simulink model "Basic_DMT"  (R2014b)
settings: Solver=FixedStepDiscrete  SolverMode=SingleTasking  StartTime=0.0  StopTime=25e-6-14e-9*24  RelTol=1e-3
PreLoadFcn:
  | userName = getenv('UserName');
  | 
  | if strcmp(userName,'Tim')
  | cd C:\Users\Tim\Documents\GitHub\MA_1\Basic_DMT
  | else
  | cd C:\Users\Tim-UML\Documents\GitHub\MA_1\Basic_DMT
  | end
InitFcn:
  | userName = getenv('UserName');
  | 
  | if strcmp(userName,'Tim')
  | cd C:\Users\Tim\Documents\GitHub\MA_1\Basic_DMT
  | else
  | cd C:\Users\Tim-UML\Documents\GitHub\MA_1\Basic_DMT
  | end
values from neighbouring files (symbols this model uses):
  a0 = 0.21194908595403703    (= 0.211949085954)    [initScript.m]
  a1 = 0.576101828091926    (= 0.576101828092)    [initScript.m]
  a2 = a0    (= 0.211949085954)    [initScript.m]
  beta = 1    [initScript.m]
  bitPerSymb = 4    [initScript.m]
  chanDownFact = Tchan/SystemPeriod    [initScript.m]
  fftLen = 16    [initScript.m]
  fftLenActive = fftLenDMT    (= 32)    [initScript.m]
  fftLenDMT = 2*fftLen    (= 32)    [initScript.m]
  GI_Active = GI_LenDMT    (= 0)    [initScript.m]
  GI_Len = 0    [initScript.m]
  GI_LenDMT = 0    [initScript.m]
  M = log2(fftLen)    [initScript.m]
  sysgenSystemPeriod = 4e-9    (= 4e-09)    [initScript.m]
  SystemPeriod = 4e-9    (= 4e-09)    [initScript.m]
  upsampleFactor = 1    [initScript.m]
  usedSubCar = 14    [initScript.m]
undefined symbols (not defined in the file or in its folder): bitCount, get, modu_mode, Tb, Ts
libraries: xbsIndex_r4 x822, commdigbbndam3 x59, simulink x42, dspsigops x7, commrandsrc2 x6, dspbuff3 x4, dspxfrm3 x3, dspswit3 x2, commseqgen2 x1, dsparch4 x1, commutil2 x1, dspsnks4 x1
(part 8 of 10)

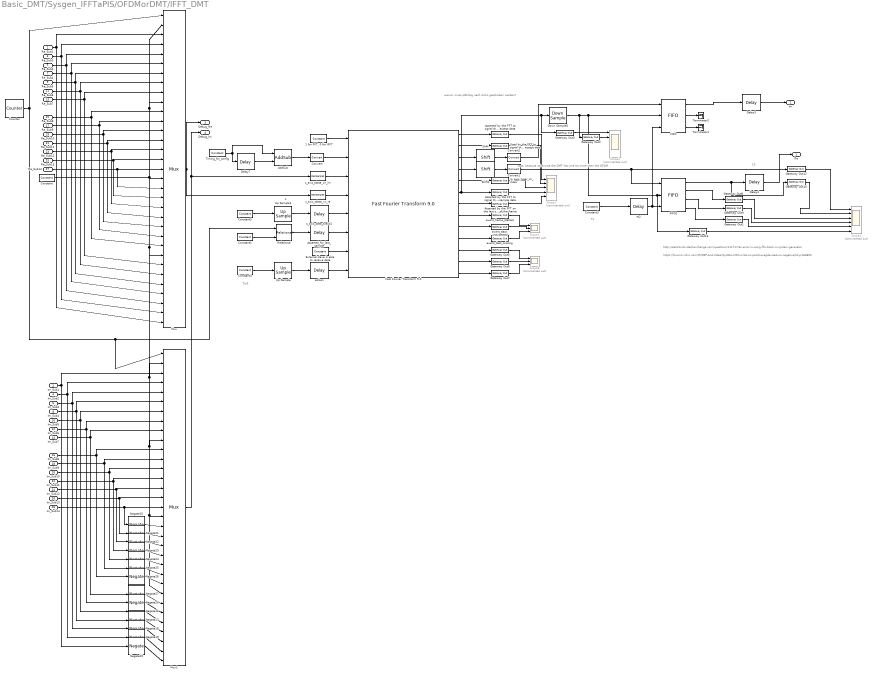
== system Basic_DMT/Sysgen_IFFTaPIS/OFDMorDMT/IFFT_DMT ==
  note: https://forums.xilinx.com/t5/DSP-and-Video/SysGen-FIFO-write-on-positive-egde-read-on-negative/td-p/168800
  note: http://electronics.stackexchange.com/questions/111717/an-error-in-using-fifo-block-in-system-generator
  note: 10
  note: warum muss plötzlicg nach öinks geschoben werden?
  note: cast, because otherwise the DMT has one bit more then the OFDM
  note: Ts
  note: 6
  note: Ts/3
  Re_Sub1 : Inport
  Im_Sub1 : Inport  Port=2
  Re_Sub2 : Inport  Port=3
  Im_Sub2 : Inport  Port=4
  Re_Sub3 : Inport  Port=5
  Im_Sub3 : Inport  Port=6
  Re_Sub4 : Inport  Port=7
  Im_Sub4 : Inport  Port=8
  Re_Sub5 : Inport  Port=9
  Im_Sub5 : Inport  Port=10
  Re_Sub6 : Inport  Port=11
  Im_Sub6 : Inport  Port=12
  Re_Sub7 : Inport  Port=13
  Im_Sub7 : Inport  Port=14
  Re_Sub8 : Inport  Port=15
  Im_Sub8 : Inport  Port=16
  Re_Sub9 : Inport  Port=17
  Im_Sub9 : Inport  Port=18
  Re_Sub10 : Inport  Port=19
  Im_Sub10 : Inport  Port=20
  Re_Sub11 : Inport  Port=21
  Im_Sub11 : Inport  Port=22
  Re_Sub12 : Inport  Port=23
  Im_Sub12 : Inport  Port=24
  Re_Sub13 : Inport  Port=25
  Im_Sub13 : Inport  Port=26
  Re_Sub14 : Inport  Port=27
  Im_Sub14 : Inport  Port=28
  "1 for FFT, 0 for IFFT " : xbsIndex_r4/Constant  const=0  gui_display_data_type=Fixed-point  arith_type=Unsigned  n_bits=1  bin_pt=0  preci_type=Single  exp_width=8  frac_width=24  explicit_period=on  period=Ts  equ=P=C  opselect=C  inp2=PCIN>>17  opr=+  inp1=P  carry=CIN  dbl_ovrd=off  block_type=constant
  AddSub : xbsIndex_r4/AddSub  mode=Subtraction  use_carryin=off  use_carryout=off  en=off  latency=0  precision=User Defined  arith_type=Unsigned  n_bits=1  bin_pt=0  quantization=Truncate  overflow=Wrap  use_behavioral_HDL=off  hw_selection=Fabric  pipelined=off  dbl_ovrd=off  block_type=addsub
  "Asserted by the FFT on the last sample of the frame " : xbsIndex_r4/Gateway Out  inherit_from_input=off  hdl_port=off  rows=1  columns=1  UseAsDAC=off  DACChannel='1'  interface=None  automatic_assignment=on  address_offset=hex2dec('00')  intf_description=''  timing_constraint=None  locs_specified=off  LOCs={}  io_standard={}  block_type=gatewayout
  "Asserted by the FFT to signal that it is ready to accept data " : xbsIndex_r4/Gateway Out  inherit_from_input=off  hdl_port=off  rows=1  columns=1  UseAsDAC=off  DACChannel='1'  interface=None  automatic_assignment=on  address_offset=hex2dec('00')  intf_description=''  timing_constraint=None  locs_specified=off  LOCs={}  io_standard={}  block_type=gatewayout
  Asserted by the FFT to signal that it is ready to provide sample data : xbsIndex_r4/Gateway Out  inherit_from_input=off  hdl_port=off  rows=1  columns=1  UseAsDAC=off  DACChannel='1'  interface=None  automatic_assignment=on  address_offset=hex2dec('00')  intf_description=''  timing_constraint=None  locs_specified=off  LOCs={}  io_standard={}  block_type=gatewayout
  Asserted_for_last_sample : xbsIndex_r4/Delay  rst=off  infoeditControl=Selection of Reset will increase slice count due to use of real FFs and instead of SRLs  en=off  latency=1  reg_retiming=off  dbl_ovrd=off  block_type=delay
  Constant : xbsIndex_r4/Constant  const=0  gui_display_data_type=Fixed-point  arith_type=Signed (2's comp)  n_bits=bitCount  bin_pt=fracLen  preci_type=Single  exp_width=8  frac_width=24  explicit_period=on  period=Ts*usedSubCar*bitPerSymb  equ=P=C  opselect=C  inp2=PCIN>>17  opr=+  inp1=P  carry=CIN  dbl_ovrd=off  block_type=constant
  Constant1 : xbsIndex_r4/Constant  const=fftLenDMT-1  gui_display_data_type=Fixed-point  arith_type=Unsigned  n_bits=5  bin_pt=0  preci_type=Single  exp_width=8  frac_width=24  explicit_period=on  period=Ts*usedSubCar*bitPerSymb/fftLenDMT  equ=P=C  opselect=C  inp2=PCIN>>17  opr=+  inp1=P  carry=CIN  dbl_ovrd=off  block_type=constant
  Constant3 : xbsIndex_r4/Constant  const=1  gui_display_data_type=Boolean  arith_type=Boolean  n_bits=1  bin_pt=0  preci_type=Single  exp_width=8  frac_width=24  explicit_period=on  period=Ts*usedSubCar*bitPerSymb/fftLenDMT  equ=P=C  opselect=C  inp2=PCIN>>17  opr=+  inp1=P  carry=CIN  dbl_ovrd=off  block_type=constant
  Constant4 : xbsIndex_r4/Constant  const=1  gui_display_data_type=Boolean  arith_type=Boolean  n_bits=1  bin_pt=0  preci_type=Single  exp_width=8  frac_width=24  explicit_period=on  period=sysgenSystemPeriod*2  equ=P=C  opselect=C  inp2=PCIN>>17  opr=+  inp1=P  carry=CIN  dbl_ovrd=off  block_type=constant
  Constant5 : xbsIndex_r4/Constant  const=1  gui_display_data_type=Boolean  arith_type=Boolean  n_bits=1  bin_pt=0  preci_type=Single  exp_width=8  frac_width=24  explicit_period=on  period=Ts*usedSubCar*bitPerSymb/fftLenDMT  equ=P=C  opselect=C  inp2=PCIN>>17  opr=+  inp1=P  carry=CIN  dbl_ovrd=off  block_type=constant
  Convert : xbsIndex_r4/Convert  gui_display_data_type=Boolean  arith_type=Boolean  n_bits=1  bin_pt=0  float_type=Single  exp_bits=8  fraction_bits=24  quantization=Truncate  overflow=Wrap  en=off  latency=1  pipeline=off  dbl_ovrd=off  block_type=convert
  Convert1 : xbsIndex_r4/Convert  gui_display_data_type=Fixed-point  arith_type="Signed  (2's comp)"  n_bits=bitCount+log2(fftLen)+1  bin_pt=fracLen  float_type=Single  exp_bits=8  fraction_bits=24  quantization=Truncate  overflow=Wrap  en=off  latency=0  pipeline=off  dbl_ovrd=off  block_type=convert
  Convert2 : xbsIndex_r4/Convert  gui_display_data_type=Fixed-point  arith_type="Signed  (2's comp)"  n_bits=bitCount+log2(fftLen)+1  bin_pt=fracLen  float_type=Single  exp_bits=8  fraction_bits=24  quantization="Round  (unbiased: +/- Inf)"  overflow=Saturate  en=off  latency=0  pipeline=off  dbl_ovrd=off  block_type=convert
  Counter : xbsIndex_r4/Counter  cnt_type=Count Limited  cnt_to=fftLenDMT-1  operation=Up  start_count=0  cnt_by_val=1  arith_type=Unsigned  n_bits=log2(fftLenDMT)  bin_pt=0  load_pin=off  rst=off  en=off  explicit_period=on  period=Ts*usedSubCar*bitPerSymb/fftLenDMT  use_behavioral_HDL=off  implementation=Fabric  dbl_ovrd=off  block_type=counter
  Delay4 : xbsIndex_r4/Delay  rst=off  infoeditControl=Selection of Reset will increase slice count due to use of real FFs and instead of SRLs  en=off  latency=11  reg_retiming=off  dbl_ovrd=off  block_type=delay
  Delay5 : xbsIndex_r4/Delay  rst=off  infoeditControl=Selection of Reset will increase slice count due to use of real FFs and instead of SRLs  en=off  latency=11  reg_retiming=off  dbl_ovrd=off  block_type=delay
  Delay7 : xbsIndex_r4/Delay  rst=off  infoeditControl=Selection of Reset will increase slice count due to use of real FFs and instead of SRLs  en=off  latency=1  reg_retiming=off  dbl_ovrd=off  block_type=delay
  Down Sample5 : xbsIndex_r4/Down Sample  sample_ratio=2  sample_phase=First Value of Frame  en=off  rst=off  latency=0  dbl_ovrd=off  block_type=dsamp
  "Externel slave is able to receive data " : xbsIndex_r4/Constant  const=1  gui_display_data_type=Boolean  arith_type=Boolean  n_bits=1  bin_pt=0  preci_type=Single  exp_width=8  frac_width=24  explicit_period=on  period=Ts  equ=P=C  opselect=C  inp2=PCIN>>17  opr=+  inp1=P  carry=CIN  dbl_ovrd=off  block_type=constant
  FIFO : xbsIndex_r4/FIFO  mem_type=Block RAM  performance_options=Standard_FIFO  embedded_registers=off  depth=32  percent_nbits=4  rst=off  rst_latency=1  en=off  use_dcount=off  use_percent_full_port=off  use_almost_empty=off  almost_empty_thresh=2  use_almost_full=off  almost_full_thresh=14  explicit_period=off  dbl_ovrd=off  block_type=fifo
  FIFO1 : xbsIndex_r4/FIFO  mem_type=Block RAM  performance_options=Standard_FIFO  embedded_registers=off  depth=32  percent_nbits=4  rst=off  rst_latency=1  en=off  use_dcount=off  use_percent_full_port=on  use_almost_empty=off  almost_empty_thresh=2  use_almost_full=off  almost_full_thresh=14  explicit_period=off  dbl_ovrd=off  block_type=fifo
  "Fast Fourier Transform 9.0 " : xbsIndex_r4/Fast Fourier Transform 9.0   transform_length=32  target_clock_frequency=250  target_data_throughput=50  implementation_options=pipelined_streaming_io  run_time_configurable_transform_length=off  phase_factor_width=16  scaling_options=unscaled  rounding_modes=convergent_rounding  aclken=on  aresetn=off  cyclic_prefix_insertion=off  output_ordering=natural_order  throttle_scheme=nonrealtime  xk_index=on  ovflo=off  trim_axipin_name=off  memory_options_data=block_ram  memory_options_phase_factors=block_ram  number_of_stages_using_block_ram_for_data_and_phase_factors=0  memory_options_reorder=block_ram  memory_options_hybrid=off  complex_mult_type=use_mults_resources  butterfly_type=use_xtremedsp_slices  channels=1  input_ordering=natural_order  input_width=16  ip_name=Fast Fourier Transform  ip_version=9.0  dsptool_ready=true  ipcore_usecache=true  ipcore_useipmodelcache=true  wrapper_available=true  port_translation_map={ 'aclken' => 'en', 'aresetn' => 'rst'}  data_format=fixed_point  block_type=xfft_v9_0
  Gateway Out{1..3,5..10,12..13} (11 alike) : xbsIndex_r4/Gateway Out  inherit_from_input=off  hdl_port=off  rows=1  columns=1  UseAsDAC=off  DACChannel='1'  interface=None  automatic_assignment=on  address_offset=hex2dec('00')  intf_description=''  timing_constraint=None  locs_specified=off  LOCs={}  io_standard={}  block_type=gatewayout
  Mux : xbsIndex_r4/Mux  inputs=32  en=off  latency=1  precision=Full  arith_type=Unsigned  n_bits=16  bin_pt=14  quantization=Truncate  overflow=Wrap  dbl_ovrd=off  block_type=mux
  Mux1 : xbsIndex_r4/Mux  inputs=32  en=off  latency=1  precision=Full  arith_type=Unsigned  n_bits=16  bin_pt=14  quantization=Truncate  overflow=Wrap  dbl_ovrd=off  block_type=mux
  Negate{15..28} (14 alike) : xbsIndex_r4/Negate  precision=User Defined  arith_type="Signed  (2's comp)"  n_bits=bitCount  bin_pt=fracLen  quantization="Round  (unbiased: +/- Inf)"  overflow=Saturate  en=off  latency=0  dbl_ovrd=off  block_type=negate
  Relational : xbsIndex_r4/Relational  mode=a=b  op_type=Bool  en=off  latency=0  dbl_ovrd=off  block_type=relational
  Scope1 : Scope  Commented=on  NumInputPorts=3
      settings: YMin=-5~-5~-5  YMax=5~5~5  SaveName=ScopeData32
  Scope2 : Scope  Commented=on  NumInputPorts=5
      settings: YMin=-5~-5~-5~-5~-5  YMax=5~5~5~5~5  SaveName=ScopeData33
  Scope3 : Scope  Commented=on  NumInputPorts=6
      settings: YMin=0~0~-1~-1~-1~-1  YMax=1~1~1~1~1~1  SaveName=ScopeData67
  Scope4 : Scope  Commented=on  NumInputPorts=6
      settings: YMin=-100~-100~-100~0~0~0  YMax=100~50~50~1~1~1  SaveName=ScopeData34
  Scope8 : Scope  Commented=on  NumInputPorts=3
      settings: YMin=-5~-5~-5  YMax=5~5~5  SaveName=ScopeData41
  Shift : xbsIndex_r4/Shift  shift_dir=Left  shift_bits=2  en=off  latency=0  precision=Full  arith_type="Signed  (2's comp)"  n_bits=16  bin_pt=14  quantization=Truncate  overflow=Wrap  dbl_ovrd=off  block_type=shift
  Shift1 : xbsIndex_r4/Shift  shift_dir=Left  shift_bits=2  en=off  latency=0  precision=Full  arith_type="Signed  (2's comp)"  n_bits=16  bin_pt=14  quantization=Truncate  overflow=Wrap  dbl_ovrd=off  block_type=shift
  Terminator1 : Terminator
  Terminator2 : Terminator
  Timing_for_config : xbsIndex_r4/Constant  const=1  gui_display_data_type=Fixed-point  arith_type=Unsigned  n_bits=1  bin_pt=0  preci_type=Single  exp_width=8  frac_width=24  explicit_period=on  period=Ts  equ=P=C  opselect=C  inp2=PCIN>>17  opr=+  inp1=P  carry=CIN  dbl_ovrd=off  block_type=constant
  Up Sample : xbsIndex_r4/Up Sample  sample_ratio=2  copy_samples=off  en=off  latency=0  dbl_ovrd=off  block_type=usamp
  Up Sample1 : xbsIndex_r4/Up Sample  sample_ratio=Ts*usedSubCar*bitPerSymb/fftLenDMT/sysgenSystemPeriod  copy_samples=off  en=off  latency=0  dbl_ovrd=off  block_type=usamp
  Used by the FFT to signal that it is ready to accept data : xbsIndex_r4/Gateway Out  inherit_from_input=off  hdl_port=off  rows=1  columns=1  UseAsDAC=off  DACChannel='1'  interface=None  automatic_assignment=on  address_offset=hex2dec('00')  intf_description=''  timing_constraint=None  locs_specified=off  LOCs={}  io_standard={}  block_type=gatewayout
  "aclken " : xbsIndex_r4/Delay  rst=off  infoeditControl=Selection of Reset will increase slice count due to use of real FFs and instead of SRLs  en=off  latency=1  reg_retiming=off  dbl_ovrd=off  block_type=delay
  event_frame_started : xbsIndex_r4/Gateway Out  inherit_from_input=off  hdl_port=off  rows=1  columns=1  UseAsDAC=off  DACChannel='1'  interface=None  automatic_assignment=on  address_offset=hex2dec('00')  intf_description=''  timing_constraint=None  locs_specified=off  LOCs={}  io_standard={}  block_type=gatewayout
  event_tlast_missing : xbsIndex_r4/Gateway Out  inherit_from_input=off  hdl_port=off  rows=1  columns=1  UseAsDAC=off  DACChannel='1'  interface=None  automatic_assignment=on  address_offset=hex2dec('00')  intf_description=''  timing_constraint=None  locs_specified=off  LOCs={}  io_standard={}  block_type=gatewayout
  event_tlast_unexpected : xbsIndex_r4/Gateway Out  inherit_from_input=off  hdl_port=off  rows=1  columns=1  UseAsDAC=off  DACChannel='1'  interface=None  automatic_assignment=on  address_offset=hex2dec('00')  intf_description=''  timing_constraint=None  locs_specified=off  LOCs={}  io_standard={}  block_type=gatewayout
  m_axis_tuser_xk_index : xbsIndex_r4/Gateway Out  inherit_from_input=off  hdl_port=off  rows=1  columns=1  UseAsDAC=off  DACChannel='1'  interface=None  automatic_assignment=on  address_offset=hex2dec('00')  intf_description=''  timing_constraint=None  locs_specified=off  LOCs={}  io_standard={}  block_type=gatewayout
  re2 : xbsIndex_r4/Delay  rst=off  infoeditControl=Selection of Reset will increase slice count due to use of real FFs and instead of SRLs  en=off  latency=1  reg_retiming=off  dbl_ovrd=off  block_type=delay
  s_axis_data_tvalid1 : xbsIndex_r4/Delay  rst=off  infoeditControl=Selection of Reset will increase slice count due to use of real FFs and instead of SRLs  en=off  latency=1  reg_retiming=off  dbl_ovrd=off  block_type=delay
  s_axis_tdata_xn_im : xbsIndex_r4/Reinterpret  force_arith_type=on  arith_type="Signed  (2's comp)"  force_bin_pt=on  bin_pt=bitCount-1  block_type=reinterpret
  s_axis_tdata_xn_re : xbsIndex_r4/Reinterpret  force_arith_type=on  arith_type="Signed  (2's comp)"  force_bin_pt=on  bin_pt=bitCount-1  block_type=reinterpret
  Re : Outport
  Im : Outport  Port=2
  Debug_Re : Outport  Port=3
  Debug_Im : Outport  Port=4
  wires:
  Constant/1 -> Mux/26, Mux1/2, Mux1/10, Mux1/18, Mux1/26, Mux/18, Mux/2, Mux/10
  Counter/1 -> Mux1/1, Relational/1, Mux/1
  "1 for FFT, 0 for IFFT "/1 -> "Fast Fourier Transform 9.0 "/1
  "Externel slave is able to receive data "/1 -> "Fast Fourier Transform 9.0 "/7
  "Fast Fourier Transform 9.0 "/2 -> Used by the FFT to signal that it is ready to accept data/1
  "Fast Fourier Transform 9.0 "/5 -> m_axis_tuser_xk_index/1
  "Fast Fourier Transform 9.0 "/6 -> Asserted by the FFT to signal that it is ready to provide sample data/1, Gateway Out3/1, Down Sample5/1
  s_axis_tdata_xn_im/1 -> "Fast Fourier Transform 9.0 "/3
  s_axis_tdata_xn_re/1 -> "Fast Fourier Transform 9.0 "/4
  "Fast Fourier Transform 9.0 "/3 -> Shift/1
  "Fast Fourier Transform 9.0 "/4 -> Shift1/1
  Mux1/1 -> Debug_Im/1, s_axis_tdata_xn_im/1
  Mux/1 -> s_axis_tdata_xn_re/1, Debug_Re/1
  AddSub/1 -> Convert/1
  Timing_for_config/1 -> Delay7/1, AddSub/1
  Delay7/1 -> AddSub/2
  Convert/1 -> "Fast Fourier Transform 9.0 "/2
  Relational/1 -> Asserted_for_last_sample/1
  Constant1/1 -> Relational/2
  Asserted_for_last_sample/1 -> "Fast Fourier Transform 9.0 "/6
  "Fast Fourier Transform 9.0 "/10 -> event_tlast_missing/1
  "Fast Fourier Transform 9.0 "/11 -> Gateway Out5/1
  "Fast Fourier Transform 9.0 "/12 -> Gateway Out6/1
  "Fast Fourier Transform 9.0 "/13 -> Gateway Out7/1
  "Fast Fourier Transform 9.0 "/9 -> event_tlast_unexpected/1
  "Fast Fourier Transform 9.0 "/8 -> event_frame_started/1
  "Fast Fourier Transform 9.0 "/1 -> "Asserted by the FFT to signal that it is ready to accept data "/1
  Gateway Out6/1 -> Scope8/2
  Gateway Out7/1 -> Scope8/3
  Gateway Out5/1 -> Scope8/1
  event_tlast_unexpected/1 -> Scope1/2
  event_frame_started/1 -> Scope1/1
  event_tlast_missing/1 -> Scope1/3
  Asserted by the FFT to signal that it is ready to provide sample data/1 -> Scope2/4
  m_axis_tuser_xk_index/1 -> Scope2/3
  "Asserted by the FFT to signal that it is ready to accept data "/1 -> Scope2/1
  Used by the FFT to signal that it is ready to accept data/1 -> Scope2/2
  Gateway Out8/1 -> Scope4/3
  Gateway Out9/1 -> Scope4/4
  Gateway Out10/1 -> Scope4/2
  Gateway Out12/1 -> Scope4/1
  FIFO/1 -> Delay5/1
  "Fast Fourier Transform 9.0 "/7 -> "Asserted by the FFT on the last sample of the frame "/1
  Gateway Out13/1 -> Scope4/6
  "Asserted by the FFT on the last sample of the frame "/1 -> Scope2/5
  Delay4/1 -> Re/1
  Delay5/1 -> Im/1
  Convert1/1 -> FIFO1/1, Gateway Out12/1
  Convert2/1 -> FIFO/1
  Down Sample5/1 -> Gateway Out2/1, Gateway Out13/1, FIFO1/2, FIFO/2
  Up Sample/1 -> "aclken "/1
  Constant4/1 -> Up Sample/1
  "aclken "/1 -> "Fast Fourier Transform 9.0 "/8
  Up Sample1/1 -> s_axis_data_tvalid1/1
  Constant5/1 -> Up Sample1/1
  s_axis_data_tvalid1/1 -> "Fast Fourier Transform 9.0 "/5
  re2/1 -> FIFO/3, FIFO1/3
  Constant3/1 -> re2/1
  FIFO/3 -> Terminator1/1
  FIFO/2 -> Terminator2/1
  FIFO1/3 -> Gateway Out9/1
  FIFO1/4 -> Gateway Out1/1
  Gateway Out1/1 -> Scope4/5
  Re_Sub14/1 -> Mux/19, Mux/17
  Re_Sub13/1 -> Mux/20, Mux/16
  Re_Sub12/1 -> Mux/21, Mux/15
  Re_Sub11/1 -> Mux/22, Mux/14
  Re_Sub10/1 -> Mux/23, Mux/13
  Re_Sub9/1 -> Mux/24, Mux/12
  Re_Sub8/1 -> Mux/25, Mux/11
  Re_Sub7/1 -> Mux/27, Mux/9
  Re_Sub6/1 -> Mux/28, Mux/8
  Re_Sub5/1 -> Mux/29, Mux/7
  Re_Sub4/1 -> Mux/30, Mux/6
  Re_Sub3/1 -> Mux/31, Mux/5
  Re_Sub2/1 -> Mux/32, Mux/4
  Re_Sub1/1 -> Mux/33, Mux/3
  Im_Sub1/1 -> Negate20/1, Mux1/3
  Im_Sub2/1 -> Negate19/1, Mux1/4
  Im_Sub3/1 -> Negate18/1, Mux1/5
  Im_Sub4/1 -> Negate17/1, Mux1/6
  Im_Sub5/1 -> Negate16/1, Mux1/7
  Im_Sub6/1 -> Negate28/1, Mux1/8
  Im_Sub7/1 -> Negate27/1, Mux1/9
  Im_Sub8/1 -> Negate26/1, Mux1/11
  Im_Sub9/1 -> Negate25/1, Mux1/12
  Im_Sub11/1 -> Negate23/1, Mux1/14
  Im_Sub12/1 -> Negate22/1, Mux1/15
  Im_Sub13/1 -> Negate21/1, Mux1/16
  Im_Sub14/1 -> Negate15/1, Mux1/17
  Negate15/1 -> Mux1/19
  Negate21/1 -> Mux1/20
  Negate22/1 -> Mux1/21
  Negate23/1 -> Mux1/22
  Negate24/1 -> Mux1/23
  Negate25/1 -> Mux1/24
  Negate26/1 -> Mux1/25
  Negate27/1 -> Mux1/27
  Negate28/1 -> Mux1/28
  Negate16/1 -> Mux1/29
  Negate17/1 -> Mux1/30
  Negate18/1 -> Mux1/31
  Negate19/1 -> Mux1/32
  Negate20/1 -> Mux1/33
  Im_Sub10/1 -> Negate24/1, Mux1/13
  Shift/1 -> Convert2/1
  Shift1/1 -> Convert1/1
  FIFO1/1 -> Gateway Out10/1, Delay4/1
  Gateway Out3/1 -> Scope3/1
  Gateway Out2/1 -> Scope3/2
  FIFO1/2 -> Gateway Out8/1

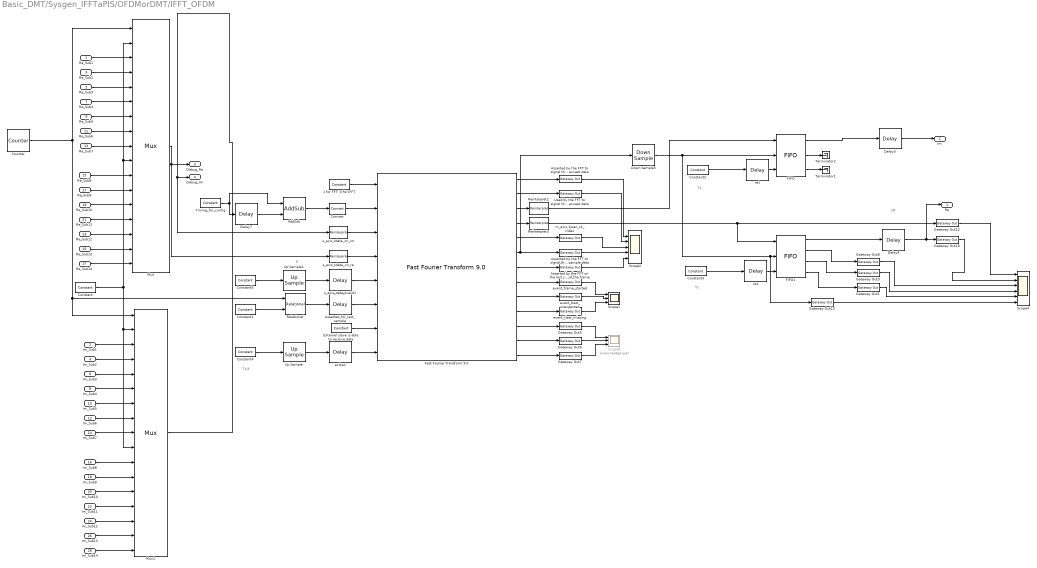
== system Basic_DMT/Sysgen_IFFTaPIS/OFDMorDMT/IFFT_OFDM ==
  note: 28
  note: Ts
  note: Ts
  note: 6
  note: Ts/3
  Re_Sub1 : Inport
  Im_Sub1 : Inport  Port=2
  Re_Sub2 : Inport  Port=3
  Im_Sub2 : Inport  Port=4
  Re_Sub3 : Inport  Port=5
  Im_Sub3 : Inport  Port=6
  Re_Sub4 : Inport  Port=7
  Im_Sub4 : Inport  Port=8
  Re_Sub5 : Inport  Port=9
  Im_Sub5 : Inport  Port=10
  Re_Sub6 : Inport  Port=11
  Im_Sub6 : Inport  Port=12
  Re_Sub7 : Inport  Port=13
  Im_Sub7 : Inport  Port=14
  Re_Sub8 : Inport  Port=15
  Im_Sub8 : Inport  Port=16
  Re_Sub9 : Inport  Port=17
  Im_Sub9 : Inport  Port=18
  Re_Sub10 : Inport  Port=19
  Im_Sub10 : Inport  Port=20
  Re_Sub11 : Inport  Port=21
  Im_Sub11 : Inport  Port=22
  Re_Sub12 : Inport  Port=23
  Im_Sub12 : Inport  Port=24
  Re_Sub13 : Inport  Port=25
  Im_Sub13 : Inport  Port=26
  Re_Sub14 : Inport  Port=27
  Im_Sub14 : Inport  Port=28
  "1 for FFT, 0 for IFFT " : xbsIndex_r4/Constant  const=0  gui_display_data_type=Fixed-point  arith_type=Unsigned  n_bits=1  bin_pt=0  preci_type=Single  exp_width=8  frac_width=24  explicit_period=on  period=Ts  equ=P=C  opselect=C  inp2=PCIN>>17  opr=+  inp1=P  carry=CIN  dbl_ovrd=off  block_type=constant
  AddSub : xbsIndex_r4/AddSub  mode=Subtraction  use_carryin=off  use_carryout=off  en=off  latency=0  precision=User Defined  arith_type=Unsigned  n_bits=1  bin_pt=0  quantization=Truncate  overflow=Wrap  use_behavioral_HDL=off  hw_selection=Fabric  pipelined=off  dbl_ovrd=off  block_type=addsub
  "Asserted by the FFT on the last sample of the frame " : xbsIndex_r4/Gateway Out  inherit_from_input=off  hdl_port=off  rows=1  columns=1  UseAsDAC=off  DACChannel='1'  interface=None  automatic_assignment=on  address_offset=hex2dec('00')  intf_description=''  timing_constraint=None  locs_specified=off  LOCs={}  io_standard={}  block_type=gatewayout
  "Asserted by the FFT to signal that it is ready to accept data " : xbsIndex_r4/Gateway Out  inherit_from_input=off  hdl_port=off  rows=1  columns=1  UseAsDAC=off  DACChannel='1'  interface=None  automatic_assignment=on  address_offset=hex2dec('00')  intf_description=''  timing_constraint=None  locs_specified=off  LOCs={}  io_standard={}  block_type=gatewayout
  Asserted by the FFT to signal that it is ready to provide sample data : xbsIndex_r4/Gateway Out  inherit_from_input=off  hdl_port=off  rows=1  columns=1  UseAsDAC=off  DACChannel='1'  interface=None  automatic_assignment=on  address_offset=hex2dec('00')  intf_description=''  timing_constraint=None  locs_specified=off  LOCs={}  io_standard={}  block_type=gatewayout
  Asserted_for_last_sample : xbsIndex_r4/Delay  rst=off  infoeditControl=Selection of Reset will increase slice count due to use of real FFs and instead of SRLs  en=off  latency=1  reg_retiming=off  dbl_ovrd=off  block_type=delay
  Constant : xbsIndex_r4/Constant  const=0  gui_display_data_type=Fixed-point  arith_type=Signed (2's comp)  n_bits=bitCount  bin_pt=fracLen  preci_type=Single  exp_width=8  frac_width=24  explicit_period=on  period=Ts*usedSubCar*bitPerSymb  equ=P=C  opselect=C  inp2=PCIN>>17  opr=+  inp1=P  carry=CIN  dbl_ovrd=off  block_type=constant
  Constant1 : xbsIndex_r4/Constant  const=fftLen-1  gui_display_data_type=Fixed-point  arith_type=Unsigned  n_bits=4  bin_pt=0  preci_type=Single  exp_width=8  frac_width=24  explicit_period=on  period=Ts*usedSubCar*bitPerSymb/fftLen  equ=P=C  opselect=C  inp2=PCIN>>17  opr=+  inp1=P  carry=CIN  dbl_ovrd=off  block_type=constant
  Constant2 : xbsIndex_r4/Constant  const=1  gui_display_data_type=Boolean  arith_type=Boolean  n_bits=1  bin_pt=0  preci_type=Single  exp_width=8  frac_width=24  explicit_period=on  period=Ts*usedSubCar*bitPerSymb/fftLen  equ=P=C  opselect=C  inp2=PCIN>>17  opr=+  inp1=P  carry=CIN  dbl_ovrd=off  block_type=constant
  Constant3 : xbsIndex_r4/Constant  const=1  gui_display_data_type=Boolean  arith_type=Boolean  n_bits=1  bin_pt=0  preci_type=Single  exp_width=8  frac_width=24  explicit_period=on  period=Ts*usedSubCar*bitPerSymb/fftLen  equ=P=C  opselect=C  inp2=PCIN>>17  opr=+  inp1=P  carry=CIN  dbl_ovrd=off  block_type=constant
  Constant4 : xbsIndex_r4/Constant  const=1  gui_display_data_type=Boolean  arith_type=Boolean  n_bits=1  bin_pt=0  preci_type=Single  exp_width=8  frac_width=24  explicit_period=on  period=sysgenSystemPeriod*2  equ=P=C  opselect=C  inp2=PCIN>>17  opr=+  inp1=P  carry=CIN  dbl_ovrd=off  block_type=constant
  Constant5 : xbsIndex_r4/Constant  const=1  gui_display_data_type=Boolean  arith_type=Boolean  n_bits=1  bin_pt=0  preci_type=Single  exp_width=8  frac_width=24  explicit_period=on  period=Ts*usedSubCar*bitPerSymb/fftLen  equ=P=C  opselect=C  inp2=PCIN>>17  opr=+  inp1=P  carry=CIN  dbl_ovrd=off  block_type=constant
  Convert : xbsIndex_r4/Convert  gui_display_data_type=Boolean  arith_type=Boolean  n_bits=1  bin_pt=0  float_type=Single  exp_bits=8  fraction_bits=24  quantization=Truncate  overflow=Wrap  en=off  latency=1  pipeline=off  dbl_ovrd=off  block_type=convert
  Counter : xbsIndex_r4/Counter  cnt_type=Count Limited  cnt_to=fftLen-1  operation=Up  start_count=0  cnt_by_val=1  arith_type=Unsigned  n_bits=log2(fftLen)  bin_pt=0  load_pin=off  rst=off  en=off  explicit_period=on  period=Ts*usedSubCar*bitPerSymb/fftLen  use_behavioral_HDL=off  implementation=Fabric  dbl_ovrd=off  block_type=counter
  Delay4 : xbsIndex_r4/Delay  rst=off  infoeditControl=Selection of Reset will increase slice count due to use of real FFs and instead of SRLs  en=off  latency=14*2+1  reg_retiming=off  dbl_ovrd=off  block_type=delay
  Delay5 : xbsIndex_r4/Delay  rst=off  infoeditControl=Selection of Reset will increase slice count due to use of real FFs and instead of SRLs  en=off  latency=14*2+1  reg_retiming=off  dbl_ovrd=off  block_type=delay
  Delay7 : xbsIndex_r4/Delay  rst=off  infoeditControl=Selection of Reset will increase slice count due to use of real FFs and instead of SRLs  en=off  latency=1  reg_retiming=off  dbl_ovrd=off  block_type=delay
  Down Sample5 : xbsIndex_r4/Down Sample  sample_ratio=2  sample_phase=First Value of Frame  en=off  rst=off  latency=0  dbl_ovrd=off  block_type=dsamp
  "Externel slave is able to receive data " : xbsIndex_r4/Constant  const=1  gui_display_data_type=Boolean  arith_type=Boolean  n_bits=1  bin_pt=0  preci_type=Single  exp_width=8  frac_width=24  explicit_period=on  period=Ts  equ=P=C  opselect=C  inp2=PCIN>>17  opr=+  inp1=P  carry=CIN  dbl_ovrd=off  block_type=constant
  FIFO : xbsIndex_r4/FIFO  mem_type=Block RAM  performance_options=Standard_FIFO  embedded_registers=off  depth=16  percent_nbits=4  rst=off  rst_latency=1  en=off  use_dcount=off  use_percent_full_port=off  use_almost_empty=off  almost_empty_thresh=2  use_almost_full=off  almost_full_thresh=14  explicit_period=off  dbl_ovrd=off  block_type=fifo
  FIFO1 : xbsIndex_r4/FIFO  mem_type=Block RAM  performance_options=Standard_FIFO  embedded_registers=off  depth=16  percent_nbits=4  rst=off  rst_latency=1  en=off  use_dcount=off  use_percent_full_port=on  use_almost_empty=off  almost_empty_thresh=2  use_almost_full=off  almost_full_thresh=14  explicit_period=off  dbl_ovrd=off  block_type=fifo
  "Fast Fourier Transform 9.0 " : xbsIndex_r4/Fast Fourier Transform 9.0   transform_length=16  target_clock_frequency=250  target_data_throughput=50  implementation_options=pipelined_streaming_io  run_time_configurable_transform_length=off  phase_factor_width=16  scaling_options=unscaled  rounding_modes=convergent_rounding  aclken=on  aresetn=off  cyclic_prefix_insertion=off  output_ordering=natural_order  throttle_scheme=nonrealtime  xk_index=on  ovflo=off  trim_axipin_name=off  memory_options_data=block_ram  memory_options_phase_factors=block_ram  number_of_stages_using_block_ram_for_data_and_phase_factors=0  memory_options_reorder=block_ram  memory_options_hybrid=off  complex_mult_type=use_mults_resources  butterfly_type=use_xtremedsp_slices  channels=1  input_ordering=natural_order  input_width=16  ip_name=Fast Fourier Transform  ip_version=9.0  dsptool_ready=true  ipcore_usecache=true  ipcore_useipmodelcache=true  wrapper_available=true  port_translation_map={ 'aclken' => 'en', 'aresetn' => 'rst'}  data_format=fixed_point  block_type=xfft_v9_0
  Gateway Out{1,5..10,12..13} (9 alike) : xbsIndex_r4/Gateway Out  inherit_from_input=off  hdl_port=off  rows=1  columns=1  UseAsDAC=off  DACChannel='1'  interface=None  automatic_assignment=on  address_offset=hex2dec('00')  intf_description=''  timing_constraint=None  locs_specified=off  LOCs={}  io_standard={}  block_type=gatewayout
  Mux : xbsIndex_r4/Mux  inputs=16  en=off  latency=1  precision=Full  arith_type=Unsigned  n_bits=16  bin_pt=14  quantization=Truncate  overflow=Wrap  dbl_ovrd=off  block_type=mux
  Mux1 : xbsIndex_r4/Mux  inputs=16  en=off  latency=1  precision=Full  arith_type=Unsigned  n_bits=16  bin_pt=14  quantization=Truncate  overflow=Wrap  dbl_ovrd=off  block_type=mux
  Reinterpret2 : xbsIndex_r4/Reinterpret  force_arith_type=on  arith_type="Signed  (2's comp)"  force_bin_pt=on  bin_pt=fracLen  block_type=reinterpret
  Reinterpret3 : xbsIndex_r4/Reinterpret  force_arith_type=on  arith_type="Signed  (2's comp)"  force_bin_pt=on  bin_pt=fracLen  block_type=reinterpret
  Relational : xbsIndex_r4/Relational  mode=a=b  op_type=Bool  en=off  latency=0  dbl_ovrd=off  block_type=relational
  Scope1 : Scope  NumInputPorts=3
      settings: YMin=-5~-5~-5  YMax=5~5~5  SaveName=ScopeData60
  Scope2 : Scope  NumInputPorts=5
      settings: YMin=-5~-5~-5~-5~-5  YMax=5~5~5~5~5  SaveName=ScopeData61
  Scope4 : Scope  NumInputPorts=6
      settings: YMin=-5~-5~-5~-5~-5~-5  YMax=5~5~5~5~5~5  SaveName=ScopeData40
  Scope8 : Scope  Commented=on  NumInputPorts=3
      settings: YMin=-5~-5~-5  YMax=5~5~5  SaveName=ScopeData59
  Terminator1 : Terminator
  Terminator2 : Terminator
  Timing_for_config : xbsIndex_r4/Constant  const=1  gui_display_data_type=Fixed-point  arith_type=Unsigned  n_bits=1  bin_pt=0  preci_type=Single  exp_width=8  frac_width=24  explicit_period=on  period=Ts  equ=P=C  opselect=C  inp2=PCIN>>17  opr=+  inp1=P  carry=CIN  dbl_ovrd=off  block_type=constant
  Up Sample : xbsIndex_r4/Up Sample  sample_ratio=2  copy_samples=off  en=off  latency=0  dbl_ovrd=off  block_type=usamp
  Up Sample1 : xbsIndex_r4/Up Sample  sample_ratio=Ts*usedSubCar*bitPerSymb/fftLen/sysgenSystemPeriod  copy_samples=off  en=off  latency=0  dbl_ovrd=off  block_type=usamp
  Used by the FFT to signal that it is ready to accept data : xbsIndex_r4/Gateway Out  inherit_from_input=off  hdl_port=off  rows=1  columns=1  UseAsDAC=off  DACChannel='1'  interface=None  automatic_assignment=on  address_offset=hex2dec('00')  intf_description=''  timing_constraint=None  locs_specified=off  LOCs={}  io_standard={}  block_type=gatewayout
  "aclken " : xbsIndex_r4/Delay  rst=off  infoeditControl=Selection of Reset will increase slice count due to use of real FFs and instead of SRLs  en=off  latency=1  reg_retiming=off  dbl_ovrd=off  block_type=delay
  event_frame_started : xbsIndex_r4/Gateway Out  inherit_from_input=off  hdl_port=off  rows=1  columns=1  UseAsDAC=off  DACChannel='1'  interface=None  automatic_assignment=on  address_offset=hex2dec('00')  intf_description=''  timing_constraint=None  locs_specified=off  LOCs={}  io_standard={}  block_type=gatewayout
  event_tlast_missing : xbsIndex_r4/Gateway Out  inherit_from_input=off  hdl_port=off  rows=1  columns=1  UseAsDAC=off  DACChannel='1'  interface=None  automatic_assignment=on  address_offset=hex2dec('00')  intf_description=''  timing_constraint=None  locs_specified=off  LOCs={}  io_standard={}  block_type=gatewayout
  event_tlast_unexpected : xbsIndex_r4/Gateway Out  inherit_from_input=off  hdl_port=off  rows=1  columns=1  UseAsDAC=off  DACChannel='1'  interface=None  automatic_assignment=on  address_offset=hex2dec('00')  intf_description=''  timing_constraint=None  locs_specified=off  LOCs={}  io_standard={}  block_type=gatewayout
  m_axis_tuser_xk_index : xbsIndex_r4/Gateway Out  inherit_from_input=off  hdl_port=off  rows=1  columns=1  UseAsDAC=off  DACChannel='1'  interface=None  automatic_assignment=on  address_offset=hex2dec('00')  intf_description=''  timing_constraint=None  locs_specified=off  LOCs={}  io_standard={}  block_type=gatewayout
  re1 : xbsIndex_r4/Delay  rst=off  infoeditControl=Selection of Reset will increase slice count due to use of real FFs and instead of SRLs  en=off  latency=1  reg_retiming=off  dbl_ovrd=off  block_type=delay
  re2 : xbsIndex_r4/Delay  rst=off  infoeditControl=Selection of Reset will increase slice count due to use of real FFs and instead of SRLs  en=off  latency=1  reg_retiming=off  dbl_ovrd=off  block_type=delay
  s_axis_data_tvalid1 : xbsIndex_r4/Delay  rst=off  infoeditControl=Selection of Reset will increase slice count due to use of real FFs and instead of SRLs  en=off  latency=1  reg_retiming=off  dbl_ovrd=off  block_type=delay
  s_axis_tdata_xn_im : xbsIndex_r4/Reinterpret  force_arith_type=on  arith_type="Signed  (2's comp)"  force_bin_pt=on  bin_pt=bitCount-1  block_type=reinterpret
  s_axis_tdata_xn_re : xbsIndex_r4/Reinterpret  force_arith_type=on  arith_type="Signed  (2's comp)"  force_bin_pt=on  bin_pt=bitCount-1  block_type=reinterpret
  Re : Outport
  Im : Outport  Port=2
  Debug_Re : Outport  Port=3
  Debug_Im : Outport  Port=4
  wires:
  Im_Sub1/1 -> Mux1/3
  Re_Sub1/1 -> Mux/3
  Counter/1 -> Mux1/1, Relational/1, Mux/1
  "1 for FFT, 0 for IFFT "/1 -> "Fast Fourier Transform 9.0 "/1
  "Externel slave is able to receive data "/1 -> "Fast Fourier Transform 9.0 "/7
  "Fast Fourier Transform 9.0 "/2 -> Used by the FFT to signal that it is ready to accept data/1
  "Fast Fourier Transform 9.0 "/5 -> m_axis_tuser_xk_index/1
  "Fast Fourier Transform 9.0 "/6 -> Asserted by the FFT to signal that it is ready to provide sample data/1, Down Sample5/1
  s_axis_tdata_xn_im/1 -> "Fast Fourier Transform 9.0 "/3
  s_axis_tdata_xn_re/1 -> "Fast Fourier Transform 9.0 "/4
  "Fast Fourier Transform 9.0 "/3 -> Reinterpret2/1
  "Fast Fourier Transform 9.0 "/4 -> Reinterpret3/1
  Mux1/1 -> s_axis_tdata_xn_im/1, Debug_Im/1
  Mux/1 -> s_axis_tdata_xn_re/1, Debug_Re/1
  AddSub/1 -> Convert/1
  Timing_for_config/1 -> Delay7/1, AddSub/1
  Delay7/1 -> AddSub/2
  Convert/1 -> "Fast Fourier Transform 9.0 "/2
  Relational/1 -> Asserted_for_last_sample/1
  Constant1/1 -> Relational/2
  Asserted_for_last_sample/1 -> "Fast Fourier Transform 9.0 "/6
  "Fast Fourier Transform 9.0 "/10 -> event_tlast_missing/1
  "Fast Fourier Transform 9.0 "/11 -> Gateway Out5/1
  "Fast Fourier Transform 9.0 "/12 -> Gateway Out6/1
  "Fast Fourier Transform 9.0 "/13 -> Gateway Out7/1
  "Fast Fourier Transform 9.0 "/9 -> event_tlast_unexpected/1
  "Fast Fourier Transform 9.0 "/8 -> event_frame_started/1
  "Fast Fourier Transform 9.0 "/1 -> "Asserted by the FFT to signal that it is ready to accept data "/1
  Gateway Out6/1 -> Scope8/2
  Gateway Out7/1 -> Scope8/3
  Gateway Out5/1 -> Scope8/1
  event_tlast_unexpected/1 -> Scope1/2
  event_frame_started/1 -> Scope1/1
  event_tlast_missing/1 -> Scope1/3
  Asserted by the FFT to signal that it is ready to provide sample data/1 -> Scope2/4
  m_axis_tuser_xk_index/1 -> Scope2/3
  "Asserted by the FFT to signal that it is ready to accept data "/1 -> Scope2/1
  Used by the FFT to signal that it is ready to accept data/1 -> Scope2/2
  Gateway Out8/1 -> Scope4/3
  Gateway Out9/1 -> Scope4/4
  Gateway Out10/1 -> Scope4/2
  Gateway Out12/1 -> Scope4/1
  re2/1 -> FIFO1/3
  FIFO1/1 -> Delay4/1
  FIFO/1 -> Delay5/1
  "Fast Fourier Transform 9.0 "/7 -> "Asserted by the FFT on the last sample of the frame "/1
  Gateway Out13/1 -> Scope4/6
  "Asserted by the FFT on the last sample of the frame "/1 -> Scope2/5
  Delay4/1 -> Gateway Out10/1, Re/1
  Delay5/1 -> Im/1
  Reinterpret3/1 -> FIFO1/1, Gateway Out12/1
  Reinterpret2/1 -> FIFO/1
  Down Sample5/1 -> Gateway Out13/1, FIFO1/2, FIFO/2
  Up Sample/1 -> "aclken "/1
  Constant4/1 -> Up Sample/1
  "aclken "/1 -> "Fast Fourier Transform 9.0 "/8
  Up Sample1/1 -> s_axis_data_tvalid1/1
  Constant5/1 -> Up Sample1/1
  s_axis_data_tvalid1/1 -> "Fast Fourier Transform 9.0 "/5
  Constant2/1 -> re1/1
  re1/1 -> FIFO/3
  Constant3/1 -> re2/1
  FIFO/3 -> Terminator1/1
  FIFO/2 -> Terminator2/1
  FIFO1/2 -> Gateway Out8/1
  FIFO1/3 -> Gateway Out9/1
  FIFO1/4 -> Gateway Out1/1
  Gateway Out1/1 -> Scope4/5
  Constant/1 -> Mux/10, Mux/2, Mux1/2, Mux1/10
  Re_Sub8/1 -> Mux/11
  Re_Sub9/1 -> Mux/12
  Re_Sub10/1 -> Mux/13
  Re_Sub11/1 -> Mux/14
  Re_Sub12/1 -> Mux/15
  Re_Sub13/1 -> Mux/16
  Re_Sub14/1 -> Mux/17
  Im_Sub2/1 -> Mux1/4
  Im_Sub3/1 -> Mux1/5
  Im_Sub4/1 -> Mux1/6
  Im_Sub5/1 -> Mux1/7
  Im_Sub6/1 -> Mux1/8
  Im_Sub7/1 -> Mux1/9
  Im_Sub8/1 -> Mux1/11
  Im_Sub9/1 -> Mux1/12
  Im_Sub10/1 -> Mux1/13
  Im_Sub11/1 -> Mux1/14
  Im_Sub12/1 -> Mux1/15
  Im_Sub13/1 -> Mux1/16
  Im_Sub14/1 -> Mux1/17
  Re_Sub2/1 -> Mux/4
  Re_Sub3/1 -> Mux/5
  Re_Sub4/1 -> Mux/6
  Re_Sub5/1 -> Mux/7
  Re_Sub6/1 -> Mux/8
  Re_Sub7/1 -> Mux/9

== system Basic_DMT/Sysgen_SIPaFFT/Delay_GI/GI_Delay_DMT ==
  note: 11
  Inp_Re : Inport
  Inp_Im : Inport  Port=2
  Delay : xbsIndex_r4/Delay  rst=off  infoeditControl=Selection of Reset will increase slice count due to use of real FFs and instead of SRLs  en=off  latency=16  reg_retiming=off  dbl_ovrd=off  block_type=delay
  Delay1 : xbsIndex_r4/Delay  rst=off  infoeditControl=Selection of Reset will increase slice count due to use of real FFs and instead of SRLs  en=off  latency=16  reg_retiming=off  dbl_ovrd=off  block_type=delay
  Out_Re : Outport
  Out_Im : Outport  Port=2
  wires:
  Inp_Re/1 -> Delay/1
  Delay/1 -> Out_Re/1
  Delay1/1 -> Out_Im/1
  Inp_Im/1 -> Delay1/1

== system Basic_DMT/Sysgen_SIPaFFT/Delay_GI/No_Delay ==
  Inp_Re : Inport
  Inp_Im : Inport  Port=2
  Out_Re : Outport
  Out_Im : Outport  Port=2
  wires:
  Inp_Re/1 -> Out_Re/1
  Inp_Im/1 -> Out_Im/1

== system Basic_DMT/Sysgen_SIPaFFT/Delay_Guard_Interval2/No_equal ==
  Re : Inport
  Im : Inport  Port=2
  MCode1 : xbsIndex_r4/MCode  mfname=Extract_Subcar_16  explicit_period=off  period=1  inputsTable={'boundInpExpr'=>['','','M','fracLen','bitCount'],'inputs'=>['x_re','x_im','M','fracLen','bitCount']}  outputsTable={'outputs'=>['y1_re','y1_im','y2_re','y2_im','y3_re','y3_im','y4_re','y4_im','y5_re','y5_im','y6_re','y6_im','y7_re','y7_im','y8_re','y8_im','y9_re','y9_im','y10_re','y10_im','y11_re','y11_im','y12_re','y12_im','y13_re','y13_im','y14_re','y14_im','y15_re','y15_im','y16_re','y16_im'],'suppressOut'=>['off','off','off','off','off','off','off','off','off','off','off','off','off','off','off','off','off','off','off','off','off','off','off','off','off','off','off','off','off','off','off','off']}  enable_stdout=off  enable_debug=off  suppress_output=on  defparams={'M',M,'fracLen',fracLen,'bitCount',bitCount}  hide_port_list={}  dbl_ovrd=off  block_type=mcode
  Re_Sub1 : Outport
  Im_Sub1 : Outport  Port=2
  Re_Sub2 : Outport  Port=3
  Im_Sub2 : Outport  Port=4
  Re_Sub3 : Outport  Port=5
  Im_Sub3 : Outport  Port=6
  Re_Sub4 : Outport  Port=7
  Im_Sub4 : Outport  Port=8
  Re_Sub5 : Outport  Port=9
  Im_Sub5 : Outport  Port=10
  Re_Sub6 : Outport  Port=11
  Im_Sub6 : Outport  Port=12
  Re_Sub7 : Outport  Port=13
  Im_Sub7 : Outport  Port=14
  Re_Sub8 : Outport  Port=15
  Im_Sub8 : Outport  Port=16
  Re_Sub9 : Outport  Port=17
  Im_Sub9 : Outport  Port=18
  Re_Sub10 : Outport  Port=19
  Im_Sub10 : Outport  Port=20
  Re_Sub11 : Outport  Port=21
  Im_Sub11 : Outport  Port=22
  Re_Sub12 : Outport  Port=23
  Im_Sub12 : Outport  Port=24
  Re_Sub13 : Outport  Port=25
  Im_Sub13 : Outport  Port=26
  Re_Sub14 : Outport  Port=27
  Im_Sub14 : Outport  Port=28
  Re_Sub15 : Outport  Port=29
  Im_Sub15 : Outport  Port=30
  Re_Sub16 : Outport  Port=31
  Im_Sub16 : Outport  Port=32
  wires:
  MCode1/1 -> Re_Sub1/1
  MCode1/2 -> Im_Sub1/1
  MCode1/3 -> Re_Sub2/1
  MCode1/4 -> Im_Sub2/1
  MCode1/5 -> Re_Sub3/1
  MCode1/6 -> Im_Sub3/1
  MCode1/7 -> Re_Sub4/1
  MCode1/8 -> Im_Sub4/1
  MCode1/9 -> Re_Sub5/1
  MCode1/10 -> Im_Sub5/1
  MCode1/11 -> Re_Sub6/1
  MCode1/12 -> Im_Sub6/1
  MCode1/13 -> Re_Sub7/1
  MCode1/14 -> Im_Sub7/1
  MCode1/15 -> Re_Sub8/1
  MCode1/16 -> Im_Sub8/1
  MCode1/18 -> Im_Sub9/1
  MCode1/17 -> Re_Sub9/1
  MCode1/19 -> Re_Sub10/1
  MCode1/20 -> Im_Sub10/1
  MCode1/21 -> Re_Sub11/1
  MCode1/22 -> Im_Sub11/1
  MCode1/23 -> Re_Sub12/1
  MCode1/24 -> Im_Sub12/1
  MCode1/25 -> Re_Sub13/1
  MCode1/26 -> Im_Sub13/1
  MCode1/27 -> Re_Sub14/1
  MCode1/28 -> Im_Sub14/1
  MCode1/29 -> Re_Sub15/1
  MCode1/30 -> Im_Sub15/1
  MCode1/31 -> Re_Sub16/1
  MCode1/32 -> Im_Sub16/1
  Im/1 -> MCode1/2
  Re/1 -> MCode1/1

== system Basic_DMT/Sysgen_SIPaFFT/Delay_Guard_Interval2/Yes_equal ==
  Re : Inport
  Im : Inport  Port=2
  MCode1 : xbsIndex_r4/MCode  mfname=Extract_Subcar_16_Equal  explicit_period=off  period=1  inputsTable={'boundInpExpr'=>['','','M','fracLen','bitCount','e1_re','e1_im','e2_re','e2_im','e3_re','e3_im','e4_re','e4_im','e5_re','e5_im','e6_re','e6_im','e7_re','e7_im','e8_re','e8_im','e9_re','e9_im','e10_re','e10_im','e11_re','e11_im','e12_re','e12_im','e13_re','e13_im','e14_re','e14_im','e15_re','e15_im','e16_re','e16_im'],'inputs'=>['x_re','x_im','M','fracLen','bitCount','e1_re','e1_im','e2_re','e2_im','e3_re','e3_im','e4_re','e4_im','e5_re','e5_im','e6_re','e6_im','e7_re','e7_im','e8_re','e8_im','e9_re','e9_im','e10_re','e10_im','e11_re','e11_im','e12_re','e12_im','e13_re','e13_im','e14_re','e14_im','e15_re','e15_im','e16_re','e16_im']}  outputsTable={'outputs'=>['y1_re','y1_im','y2_re','y2_im','y3_re','y3_im','y4_re','y4_im','y5_re','y5_im','y6_re','y6_im','y7_re','y7_im','y8_re','y8_im','y9_re','y9_im','y10_re','y10_im','y11_re','y11_im','y12_re','y12_im','y13_re','y13_im','y14_re','y14_im','y15_re','y15_im','y16_re','y16_im'],'suppressOut'=>['off','off','off','off','off','off','off','off','off','off','off','off','off','off','off','off','off','off','off','off','off','off','off','off','off','off','off','off','off','off','off','off']}  enable_stdout=off  enable_debug=off  suppress_output=on  defparams={'M',M,'fracLen',fracLen,'bitCount',bitCount,'e1_re',e1_re,'e1_im',e1_im,'e2_re',e2_re,'e2_im',e2_im,'e3_re',e3_re,'e3_im',e3_im,'e4_re',e4_re,'e4_im',e4_im,'e5_re',e5_re,'e5_im',e5_im,'e6_re',e6_re,'e6_im',e6_im,'e7_re',e7_re,'e7_im',e7_im,'e8_re',e8_re,'e8_im',e8_im,'e9_re',e9_re,'e9_im',e9_im,'e10_re',e10_re,'e10_im',e10_im,'e11_re',e11_re,'e11_im',e11_im,'e12_re',e12_re,'e12_im',e12_im,'e13_re',e13_re,'e13_im',e13_im,'e14_re',e14_re,'e14_im',e14_im,'e15_re',e15_re,'e15_im',e15_im,'e16_re',e16_re,'e16_im',e16_im}  hide_port_list={}  dbl_ovrd=off  block_type=mcode
  Re_Sub1 : Outport
  Im_Sub1 : Outport  Port=2
  Re_Sub2 : Outport  Port=3
  Im_Sub2 : Outport  Port=4
  Re_Sub3 : Outport  Port=5
  Im_Sub3 : Outport  Port=6
  Re_Sub4 : Outport  Port=7
  Im_Sub4 : Outport  Port=8
  Re_Sub5 : Outport  Port=9
  Im_Sub5 : Outport  Port=10
  Re_Sub6 : Outport  Port=11
  Im_Sub6 : Outport  Port=12
  Re_Sub7 : Outport  Port=13
  Im_Sub7 : Outport  Port=14
  Re_Sub8 : Outport  Port=15
  Im_Sub8 : Outport  Port=16
  Re_Sub9 : Outport  Port=17
  Im_Sub9 : Outport  Port=18
  Re_Sub10 : Outport  Port=19
  Im_Sub10 : Outport  Port=20
  Re_Sub11 : Outport  Port=21
  Im_Sub11 : Outport  Port=22
  Re_Sub12 : Outport  Port=23
  Im_Sub12 : Outport  Port=24
  Re_Sub13 : Outport  Port=25
  Im_Sub13 : Outport  Port=26
  Re_Sub14 : Outport  Port=27
  Im_Sub14 : Outport  Port=28
  Re_Sub15 : Outport  Port=29
  Im_Sub15 : Outport  Port=30
  Re_Sub16 : Outport  Port=31
  Im_Sub16 : Outport  Port=32
  wires:
  MCode1/1 -> Re_Sub1/1
  MCode1/2 -> Im_Sub1/1
  MCode1/3 -> Re_Sub2/1
  MCode1/4 -> Im_Sub2/1
  MCode1/5 -> Re_Sub3/1
  MCode1/6 -> Im_Sub3/1
  MCode1/7 -> Re_Sub4/1
  MCode1/8 -> Im_Sub4/1
  MCode1/9 -> Re_Sub5/1
  MCode1/10 -> Im_Sub5/1
  MCode1/11 -> Re_Sub6/1
  MCode1/12 -> Im_Sub6/1
  MCode1/13 -> Re_Sub7/1
  MCode1/14 -> Im_Sub7/1
  MCode1/15 -> Re_Sub8/1
  MCode1/16 -> Im_Sub8/1
  MCode1/18 -> Im_Sub9/1
  MCode1/17 -> Re_Sub9/1
  MCode1/19 -> Re_Sub10/1
  MCode1/20 -> Im_Sub10/1
  MCode1/21 -> Re_Sub11/1
  MCode1/22 -> Im_Sub11/1
  MCode1/23 -> Re_Sub12/1
  MCode1/24 -> Im_Sub12/1
  MCode1/25 -> Re_Sub13/1
  MCode1/26 -> Im_Sub13/1
  MCode1/27 -> Re_Sub14/1
  MCode1/28 -> Im_Sub14/1
  MCode1/29 -> Re_Sub15/1
  MCode1/30 -> Im_Sub15/1
  MCode1/31 -> Re_Sub16/1
  MCode1/32 -> Im_Sub16/1
  Im/1 -> MCode1/2
  Re/1 -> MCode1/1
